simulink model "math_pendulum"  (R2024a)
settings: Solver=VariableStepAuto  StartTime=0.0  StopTime=10.0  MaxStep=0.01  RelTol=1e-3
undefined symbols (not defined in the file or in its folder): degtorad
libraries: simulink_extras x1
settings Model: Creator=xeon_ssd  LastModifiedBy=xeon_ssd

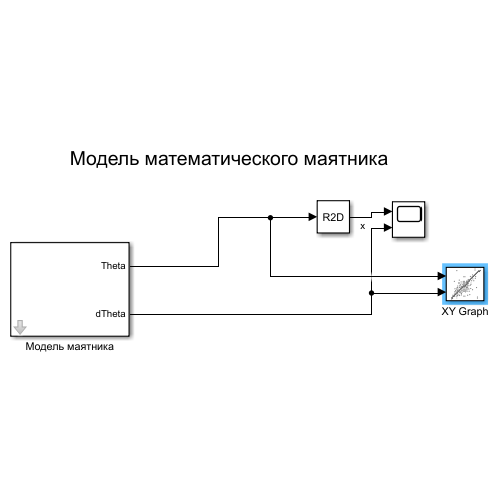
[thumbnail: Simulink's stored preview of the top-level diagram]
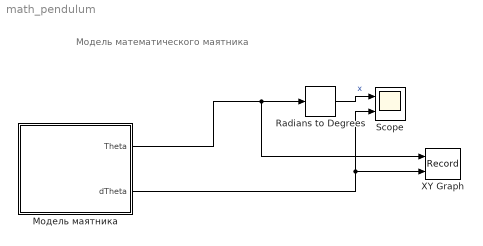
== system math_pendulum ==
  note: Модель математического маятника
  Radians to Degrees : simulink_extras/Transformations/Radians to Degrees
  Scope : Scope  NumInputPorts=2
  XY Graph : Record  FileSettingsInternal="{\"entries\":[{\"content\":{\"excelSettings\":{\"content\":{},\"type\":\"Streamout.ExcelSettings\"}},\"type\":\"Streamout.FileSettingStorage\",\"uuid\":\"\"}],\"packageUris\":[\"http:\\/\\/schema.mathworks.com\\/mf0\\/streamout_blocks\\/R2020a\"],\"version\":\"1.0\"}"  Layout=[1 1]  SignalsInternal="{\"entries\":[{\"content\":{\"signals\":[{\"content\":{\"blockPath\":[],\"dimensions\":[1],\"domain\":\"\",\"lineColor\":\"#a2142f\",\"plots\":[ 1 ],\"port\":1,\"sid\":[\"\"],\"signalID\":1,\"signalName\":\"Модель маятника:1\"},\"type\":\"RecordBlkView.Signal\",\"uuid\":\"\"},{\"content\":{\"blockPath\":[],\"dimensions\":[1],\"domain\":\"\",\"lineColor\":\"#139fff\",\"plots\":[ 1 ],\"port\":2,\"sid\":[\"\"],\"signalID\":2,\"signalName\":\"Модель маятника:2\"},\"type\":\"RecordBlkView.Signal\",\"uuid\":\"\"}]},\"type\":\"RecordBlkView.InputSignals\",\"uuid\":\"\"}],\"packageUris\":[\"http:\\/\\/schema.mathworks.com\\/mf0\\/streamout_blocks\\/R2020a\"],\"version\":\"1.0\"}"  VisualizationBindings="{\"xyplotplugin\":{\"info\":[{\"series\":[{\"bindingParametersList\":[{\"parameter\":\"X-Axis\",\"signalID\":1,\"signalName\":\"Модель маятника:1\"},{\"parameter\":\"Y-Axis\",\"signalID\":2,\"signalName\":\"Модель маятника:2\"}],\"seriesID\":0}],\"subplotID\":1}]}}"  CompatibilityTag=XY
  Модель маятника : Subsystem  mask{m=1, l=1, g=9.8, I=1, startDegree=179}
      mask prompts: m "Масса"; l "Длина подвеса"; g "Ускорение"; I "И"; startDegree "Стартовый угол"
  wires:
  Radians to Degrees/1 -> Scope/1  "x"
  Модель маятника/1(Theta) -> XY Graph/1, Radians to Degrees/1
  Модель маятника/2(dTheta) -> XY Graph/2, Scope/2

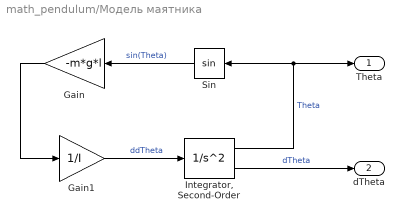
== system math_pendulum/Модель маятника ==
  Gain : Gain  Gain=-m*g*l
  Gain1 : Gain  Gain=1/I
  "Integrator, Second-Order" : SecondOrderIntegrator  ICX=degtorad(startDegree)
  Sin : Trigonometry
  Theta : Outport
  dTheta : Outport  Port=2
  wires:
  Sin/1 -> Gain/1  "sin(Theta)"
  "Integrator, Second-Order"/1 -> Theta/1, Sin/1  "Theta"
  Gain1/1 -> "Integrator, Second-Order"/1  "ddTheta"
  Gain/1 -> Gain1/1
  "Integrator, Second-Order"/2 -> dTheta/1  "dTheta"
